simulink model "boostwithPO"  (R2020b)
settings: Solver=ode23t  StartTime=0.0  StopTime=2  RelTol=1e-3
undefined symbols (not defined in the file): sigbuilder_block
libraries: powerlib x9, re_lib x1, powerlib_meascontrol x1
settings Model: Creator=shashank Pathak  LastModifiedBy=shashank Pathak

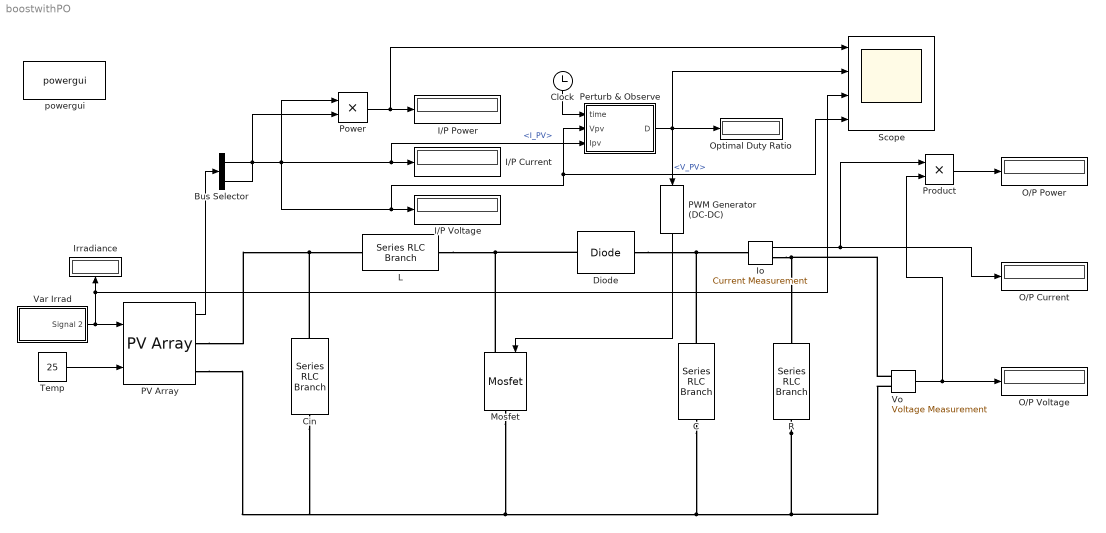
== system boostwithPO ==
  Bus Selector : BusSelector  OutputSignals=V_PV,I_PV
  C : powerlib/Elements/Series RLC Branch  LConnTagsString=__new0  RConnTagsString=__new0  BranchType=C  Resistance=1  Inductance=1e-3  SetiL0=off  InitialCurrent=0  Capacitance=3e-5  Setx0=off  InitialVoltage=0  Measurements=None
  Cin : powerlib/Elements/Series RLC Branch  LConnTagsString=__new0  RConnTagsString=__new0  BranchType=RC  Resistance=0.0001  Inductance=1.875e-4  SetiL0=off  InitialCurrent=0  Capacitance=1000e-6  Setx0=off  InitialVoltage=0  Measurements=None
  Clock : Clock
  Diode : powerlib/Power Electronics/Diode  Ron=0.001  Lon=0  Vf=0.8  IC=0  UseSnubber=0  Rs=500  Cs=250e-9  Measurements=off
  I/P Current : Display
  I/P Power : Display
  I/P Voltage : Display
  Io : powerlib/Measurements/Current Measurement  PhasorSimulation=off  OutputType=Complex  PSBequivalent=0
  Irradiance : Display
  L : powerlib/Elements/Series RLC Branch  LConnTagsString=__new0  RConnTagsString=__new0  BranchType=L  Resistance=1  Inductance=1.875e-4  SetiL0=off  InitialCurrent=0  Capacitance=1e-6  Setx0=off  InitialVoltage=0  Measurements=None
  Mosfet : powerlib/Power Electronics/Mosfet  Ron=0.1  Lon=0  Rd=0.01  Vfd=0  IC=0  Rs=1e5  Cs=inf  Measurements=off
  O/P Current : Display
  O/P Power : Display
  O/P Voltage : Display
  Optimal Duty Ratio : Display
  PV Array : re_lib/Solar/PV Array  Npar=1  Nser=1  PlotType=one module @ 25 deg.C & specified irradiances  S_vec=[ 1000 500 100 ]  Temp_C_vec="[ 45 25  ]"  ModuleName=User-defined  PlotWhenSelected=off  Pm=213.15  Ncell=60  Voc=36.3  Isc=7.84  Vm=29  Im=7.35  beta_Voc_pc=-0.36099  alpha_Isc_pc=0.102  beta_Voc=-0.13104  alpha_Isc=0.0079968  IL=7.8654  I0=2.9273e-10  nI=0.98119  Rsh=313.0553  Rs=0.39381  RobustModel=off  RobustCellTemperature=313.3991  BAL=on  Tc=1e-6  Tfilter=5e-5
  PWM Generator (DC-DC) : powerlib_meascontrol/Pulse & Signal Generators/PWM Generator (DC-DC)  Fsw=5000  Ts=10e-6
  Perturb & Observe : MATLAB Function  TreatAsAtomicUnit=on
  Power : Product
  Product : Product
  R : powerlib/Elements/Series RLC Branch  LConnTagsString=__new0  RConnTagsString=__new0  BranchType=R  Resistance=100  Inductance=1e-3  SetiL0=off  InitialCurrent=0  Capacitance=1e-6  Setx0=off  InitialVoltage=0  Measurements=None
  Scope : Scope  NumInputPorts=4
  Temp : Constant  Value=25
  Var Irrad : Subsystem  Tag=STV Subsys  LoadFcn=sigbuilder_block('load');  StartFcn=sigbuilder_block('start');  StopFcn=sigbuilder_block('stop');  ClipboardFcn=sigbuilder_block('clipboard');  mask(Sigbuilder block){tuvar=[0:10]}
      mask help: Simulink:masks:SigbuilderBlock_MD
      mask init:
      | if ~strcmp(get_param(bdroot(gcbh),'SimulationStatus'),'stopped') tuvar = sigbuilder_block('maskInit'); end
      settings: CopyFcn=sigbuilder_block('copy');  DeleteFcn=sigbuilder_block('delete');  ModelCloseFcn=sigbuilder_block('modelClose');  PreSaveFcn=sigbuilder_block('preSave');  PauseFcn=sigbuilder_block('pause');  ContinueFcn=sigbuilder_block('continue');  NameChangeFcn=sigbuilder_block('namechange');  OpenFcn=sigbuilder_block('open',[381.6 96.6 550.8 400.2 ]);  CloseFcn=sigbuilder_block('close');
      mask Display: plot(0, 0, 100, 100,[2, 2, 32, 32, 2], [68, 8, 8, 68, 68],[32, 2], [38, 38], [32, 19, 2],[53, 60, 44], [32, 17, 17, 2],[16, 16, 31, 31]);txt = getActiveGroup(gcbh);text(2, 100, txt,'verticalAlignment', 'top');
  Vo : powerlib/Measurements/Voltage Measurement  PhasorSimulation=off  OutputType=Complex  PSBequivalent=0
  powergui : powerlib/powergui  Priority=1  SimulationMode=Discrete  SampleTime=1e-6  frequency=60  Iterations=50  frequencyindice=0  Pbase=100e6  ErrMax=1e-4  UnitsV=kV  UnitsW=MW  buscounter=0  FunctionMessages=off  echomessages=off  EnableUseOfTLC=off  CurrentSourceSwitches=off  DisableSnubberDevices=off  DisableRonSwitches=off  DisableVfSwitches=off  DisplayEquations=off  AutomaticDiscreteSolvers=off  SolverType=Tustin/Backward Euler (TBE)  Interpol=off  ExternalGateDelay=off  methode=off  Ts=100  x0status=blocks  SPID=on  SwTol=0  HookPort=off  NonlinearTolerance=1e-4  nMaxIteration=100  ContinueOnMaxIteration=off  RestoreLinks=warning  ResistiveCurrentMeasurement=off  Frange=[0:2:500]  Ylog=off  Xlog=on  ShowGrid=off  save=off  variable=ZData  structure=0  ZoomFFT=off  StartTime=0.0  cycles=1  DisplayStyle=1  fundamental=60  FreqAxis=off  MaxFrequency=1000  frequencyindicesteady=1  RmsSteady=1  display=off
  wires:
  Vo/1 -> Product/2, O/P Voltage/1
  Temp/1 -> PV Array/2
  Product/1 -> O/P Power/1
  PV Array/1 -> Bus Selector/1
  Bus Selector/1 -> Scope/4, Perturb & Observe/2(Vpv), I/P Voltage/1, Power/1  "<V_PV>"
  Bus Selector/2 -> Power/2, Perturb & Observe/3(Ipv), I/P Current/1  "<I_PV>"
  Power/1 -> Scope/1, I/P Power/1
  Io/1 -> O/P Current/1, Product/1
  PWM Generator (DC-DC)/1 -> Mosfet/1
  Perturb & Observe/1(D) -> Optimal Duty Ratio/1, Scope/2, PWM Generator (DC-DC)/1
  Clock/1 -> Perturb & Observe/1(time)
  Var Irrad/1(Signal 2) -> PV Array/1, Scope/3, Irradiance/1
  connections:
  C/LConn1 -- Diode/RConn1 -- Io/LConn1
  R/RConn1 -- Vo/LConn2 -- Mosfet/RConn1 -- PV Array/RConn2 -- Cin/RConn1 -- C/RConn1
  L/RConn1 -- Diode/LConn1 -- Mosfet/LConn1
  PV Array/RConn1 -- Cin/LConn1 -- L/LConn1
  Io/RConn1 -- R/LConn1 -- Vo/LConn1

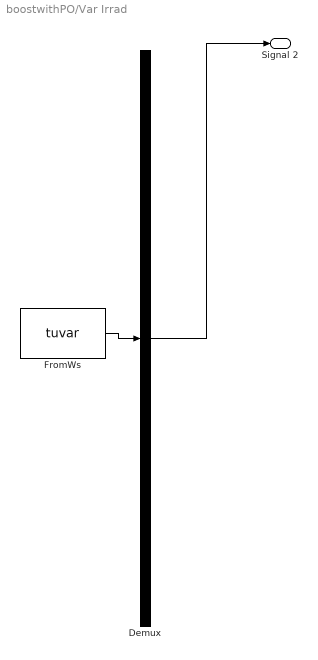
== system boostwithPO/Var Irrad ==
  Demux : Demux  Tag=STV Demux  Outputs=1
      settings: DisplayOption=none
  FromWs : FromWorkspace  Tag=STV FromWs  VariableName=tuvar
      SigBuilderData=|
      | common.afterFinalStr = 'Extrapolate'
      | common.sampleTime = 0
      | dataSet.timeRange = [0 2]
      | dataSet.name = 'Group 1'
      | sbobj.Groups.Name = 'Group 1'
      | sbobj.Groups.Signals.Name = 'Signal 2'
      | sbobj.Groups.Signals.XData = [0 0.5 0.5 1 1 1.5 1.5 2]
      | sbobj.Groups.Signals.YData = [1000 1000 600 600 800 800 1000 1000]
      | sbobj.Groups.TimeRange = [0 2]
  Signal 2 : Outport  Tag=STV Outport
  wires:
  FromWs/1 -> Demux/1
  Demux/1 -> Signal 2/1

== matlab function boostwithPO/Perturb & Observe ==
  data: time input; Vpv input; D output; Ipv input
function D = PO(time, Vpv, Ipv)

persistent Dprev Vprev Pprev prevTime

if isempty(prevTime)
    prevTime = 0;
    Dprev = 0.5;
    Vprev = Vpv;
    Pprev = Vpv * Ipv;
end

dT = time - prevTime;
delD = 0.01;
timeStep = 0.01;

if dT >= timeStep && time >= 0.1
    Ppv = Vpv * Ipv;
    dP = Ppv - Pprev;
    dV = Vpv - Vprev;
    if dP ~= 0
        if dP > 0
            if dV > 0
                % left side of MPP
                D = Dprev - delD;
            else
                % right side of MPP
                D = Dprev + delD;
            end
        else
            if dV > 0
                % right side of MPP
                D = Dprev + delD;
            else
                % left side of MPP
                D = Dprev - delD;
            end
        end
    else
        % MPP reached
        D = Dprev;
    end
    % Store current values in the previous variables
    Dprev = D;
    prevTime = time;
    Pprev = Ppv;
    Vprev = Vpv;
else
    % MPPT is not engaged
    D = Dprev;
end

end
